simulink model "main_sim"  (R2021b)
settings: Solver=VariableStepAuto  StartTime=0.0  StopTime=10.0  RelTol=1e-3
settings Model: Creator=Alex Zhen  LastModifiedBy=Alex Zhen

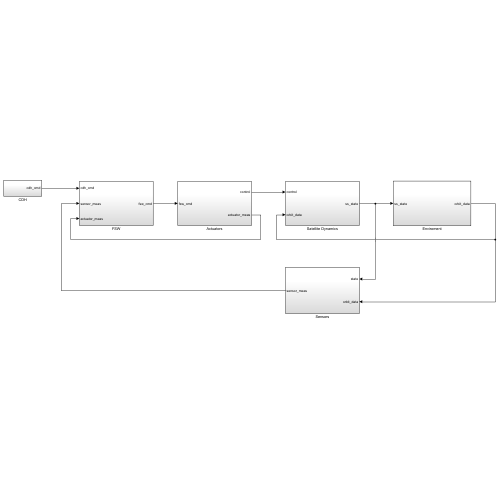
[thumbnail: Simulink's stored preview of the top-level diagram]
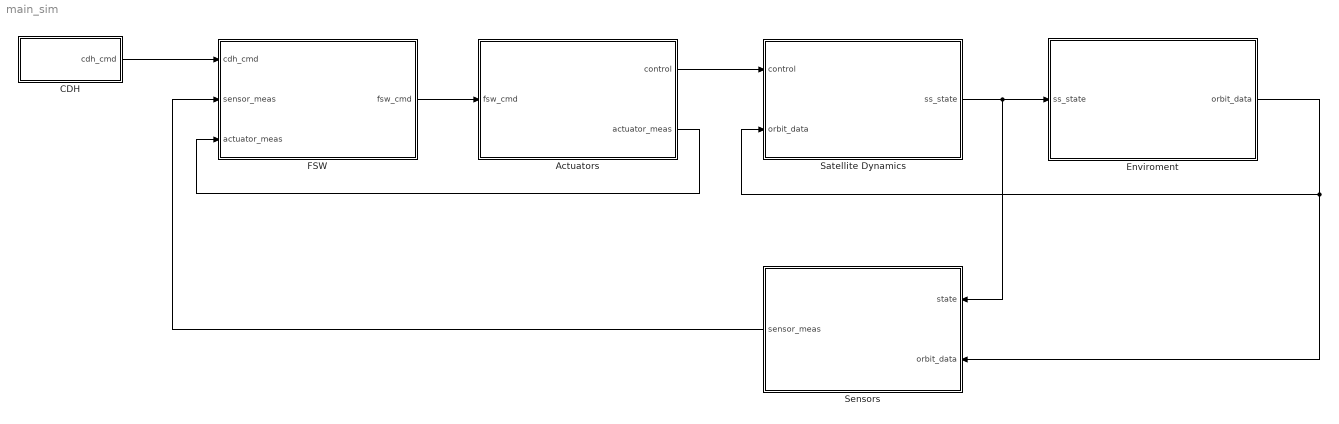
== system main_sim ==
  Actuators : Subsystem
  CDH : Subsystem
  Enviroment : Subsystem
  FSW : Subsystem
  Satellite Dynamics : Subsystem
  Sensors : Subsystem
  wires:
  FSW/1(fsw_cmd) -> Actuators/1(fsw_cmd)
  Actuators/1(control) -> Satellite Dynamics/1(control)
  Actuators/2(actuator_meas) -> FSW/3(actuator_meas)
  Sensors/1(sensor_meas) -> FSW/2(sensor_meas)
  Satellite Dynamics/1(ss_state) -> Enviroment/1(ss_state), Sensors/1(state)
  Enviroment/1(orbit_data) -> Sensors/2(orbit_data), Satellite Dynamics/2(orbit_data)
  CDH/1(cdh_cmd) -> FSW/1(cdh_cmd)

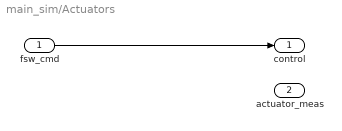
== system main_sim/Actuators ==
  fsw_cmd : Inport
  control : Outport
  actuator_meas : Outport  Port=2
  wires:
  fsw_cmd/1 -> control/1

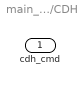
== system main_sim/CDH ==
  cdh_cmd : Outport
  wires:
  ? -> cdh_cmd/1

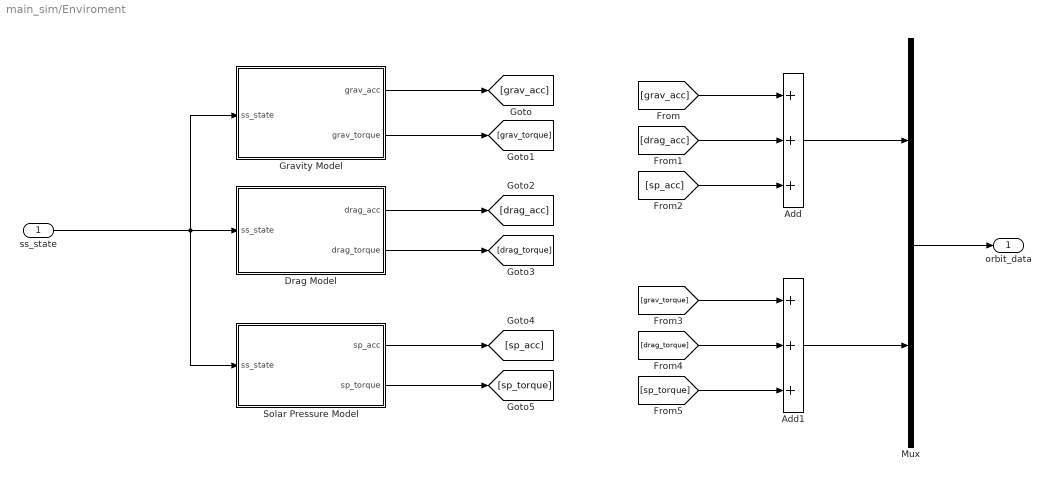
== system main_sim/Enviroment ==
  ss_state : Inport
  Add : Sum  Inputs=+++
  Add1 : Sum  Inputs=+++
  Drag Model : Subsystem
  Gravity Model : Subsystem
  Mux : Mux  Inputs=2
  Solar Pressure Model : Subsystem
  orbit_data : Outport
  wires:
  ss_state/1 -> Solar Pressure Model/1(ss_state), Drag Model/1(ss_state), Gravity Model/1(ss_state)
  Gravity Model/1(grav_acc) -> [grav_acc]
  Gravity Model/2(grav_torque) -> [grav_torque]
  Solar Pressure Model/1(sp_acc) -> [sp_acc]
  Solar Pressure Model/2(sp_torque) -> [sp_torque]
  Drag Model/2(drag_torque) -> [drag_torque]
  Drag Model/1(drag_acc) -> [drag_acc]
  [grav_acc] -> Add/1
  [drag_acc] -> Add/2
  [sp_acc] -> Add/3
  [grav_torque] -> Add1/1
  [drag_torque] -> Add1/2
  [sp_torque] -> Add1/3
  Add/1 -> Mux/1
  Add1/1 -> Mux/2
  Mux/1 -> orbit_data/1

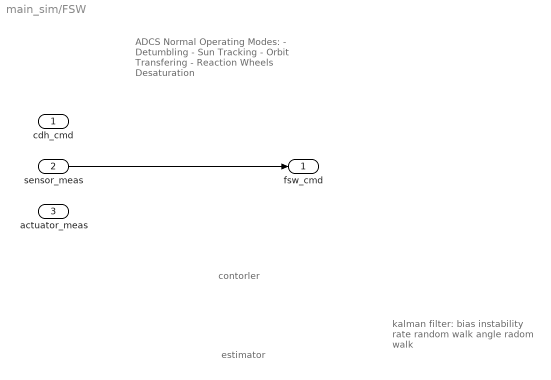
== system main_sim/FSW ==
  note: kalman filter:
      | bias instability
      | rate random walk
      | angle radom walk
  note: estimator
  note: contorler
  note: ADCS Normal Operating Modes:
      | - Detumbling
      | - Sun Tracking
      | - Orbit Transfering
      | - Reaction Wheels Desaturation
  cdh_cmd : Inport
  sensor_meas : Inport  Port=2
  actuator_meas : Inport  Port=3
  fsw_cmd : Outport
  wires:
  sensor_meas/1 -> fsw_cmd/1

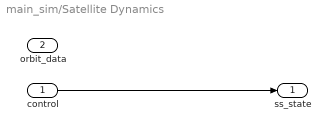
== system main_sim/Satellite Dynamics ==
  control : Inport
  orbit_data : Inport  Port=2
  ss_state : Outport
  wires:
  control/1 -> ss_state/1

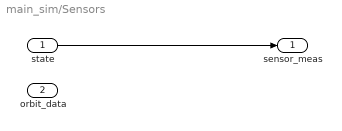
== system main_sim/Sensors ==
  state : Inport
  orbit_data : Inport  Port=2
  sensor_meas : Outport
  wires:
  state/1 -> sensor_meas/1

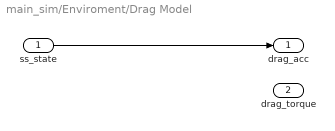
== system main_sim/Enviroment/Drag Model ==
  ss_state : Inport
  drag_acc : Outport
  drag_torque : Outport  Port=2
  wires:
  ss_state/1 -> drag_acc/1

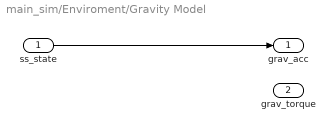
== system main_sim/Enviroment/Gravity Model ==
  ss_state : Inport
  grav_acc : Outport
  grav_torque : Outport  Port=2
  wires:
  ss_state/1 -> grav_acc/1

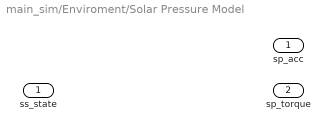
== system main_sim/Enviroment/Solar Pressure Model ==
  ss_state : Inport
  sp_acc : Outport
  sp_torque : Outport  Port=2
  wires:
  ? -> sp_acc/1
